simulink model "Longitudinal_Discrete_Servo_OutputFeedback"  (R2018b)
settings: Solver=VariableStepAuto  StartTime=0.0  StopTime=50  RelTol=1e-3
undefined symbols (not defined in the file): Gxd_A_obs, Gxd_B_obs, Gxd_C_obs, K0_X, K_X, KGe_X, t_samp
libraries: simulink x1
settings Model: Creator=Henrique  LastModifiedBy=Henrique

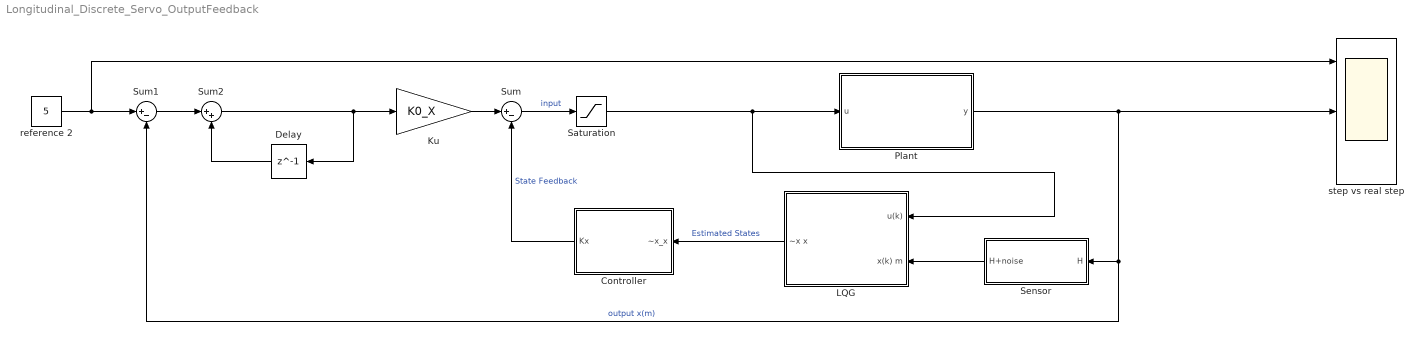
== system Longitudinal_Discrete_Servo_OutputFeedback ==
  "Controller " : Subsystem
  Delay : Delay  DelayLength=1  InitialCondition=0
  Ku : Gain  Gain=K0_X
  LQG : Subsystem
  Plant : Subsystem
  Saturation : Saturate  UpperLimit=2  LowerLimit=-1.2
  Sensor : Subsystem
  Sum : Sum  Inputs=|+-
  Sum1 : Sum  Inputs=|+-
  Sum2 : Sum  Inputs=|++
  reference 2 : Constant  Value=5
  "step vs real step " : Scope  NumInputPorts=3
  wires:
  LQG/1("~x x ") -> "Controller "/1(~x_x)  "Estimated States"
  Sum/1 -> Saturation/1  "input"
  "Controller "/1(Kx) -> Sum/2  "State Feedback"
  Plant/1("y ") -> "step vs real step "/2, Sensor/1(H), Sum1/2  "output x(m)"
  Saturation/1 -> Plant/1("u "), LQG/1(u(k))
  Sensor/1(H+noise) -> LQG/2(x(k) m)
  reference 2/1 -> Sum1/1, "step vs real step "/1
  Sum1/1 -> Sum2/1
  Sum2/1 -> Ku/1, Delay/1
  Ku/1 -> Sum/1
  Delay/1 -> Sum2/2

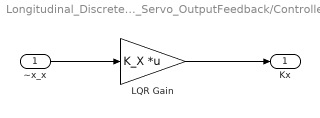
== system Longitudinal_Discrete_Servo_OutputFeedback/Controller  ==
  ~x_x : Inport
  "LQR Gain " : Gain  Gain=K_X  Multiplication=Matrix(K*u) (u vector)
  Kx : Outport
  wires:
  ~x_x/1 -> "LQR Gain "/1
  "LQR Gain "/1 -> Kx/1

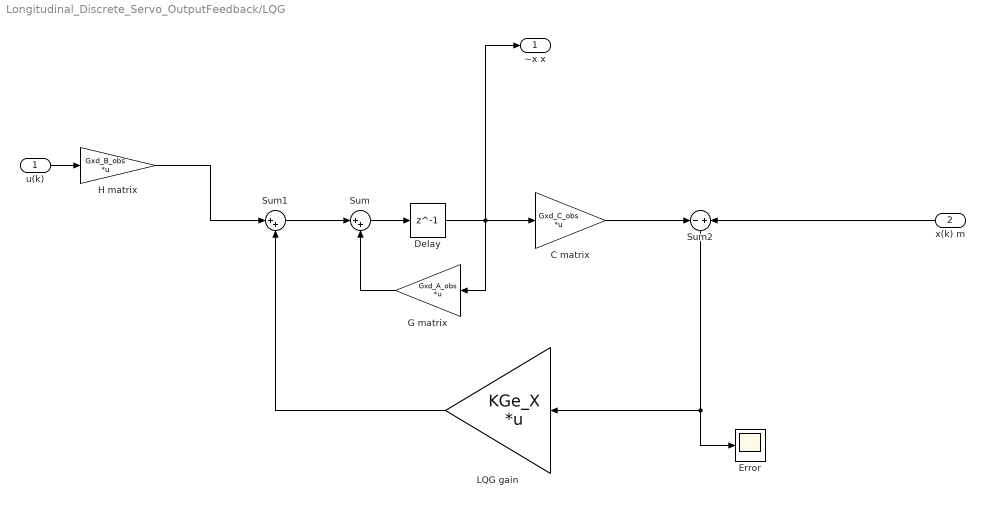
== system Longitudinal_Discrete_Servo_OutputFeedback/LQG ==
  u(k) : Inport
  x(k) m : Inport  Port=2
  C matrix : Gain  Gain=Gxd_C_obs  Multiplication=Matrix(K*u)
  Delay : Delay  DelayLength=1  InitialCondition=0  SampleTime=t_samp
  Error : Scope
  G matrix : Gain  Gain=Gxd_A_obs  Multiplication=Matrix(K*u)
  H matrix : Gain  Gain=Gxd_B_obs  Multiplication=Matrix(K*u)
  LQG gain : Gain  Gain=KGe_X  Multiplication=Matrix(K*u)
  Sum : Sum  Inputs=|++
  Sum1 : Sum  Inputs=|++
  Sum2 : Sum  Inputs=-+
  "~x x " : Outport
  wires:
  C matrix/1 -> Sum2/1
  x(k) m/1 -> Sum2/2
  H matrix/1 -> Sum1/1
  Sum/1 -> Delay/1
  u(k)/1 -> H matrix/1
  G matrix/1 -> Sum/2
  Sum2/1 -> Error/1, LQG gain/1
  LQG gain/1 -> Sum1/2
  Delay/1 -> "~x x "/1, G matrix/1, C matrix/1
  Sum1/1 -> Sum/1

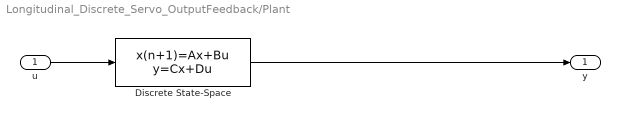
== system Longitudinal_Discrete_Servo_OutputFeedback/Plant ==
  "u " : Inport
  Discrete State-Space : DiscreteStateSpace  A=Gxd_A_obs  B=Gxd_B_obs  C=Gxd_C_obs  D=0  SampleTime=t_samp
  "y " : Outport
  wires:
  "u "/1 -> Discrete State-Space/1
  Discrete State-Space/1 -> "y "/1

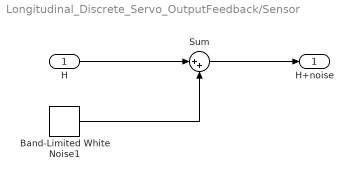
== system Longitudinal_Discrete_Servo_OutputFeedback/Sensor ==
  H : Inport
  Band-Limited White Noise1 : simulink/Sources/Band-Limited White Noise  Cov=.000001  Ts=0.1  seed=[124123]
  Sum : Sum  Inputs=|++
  H+noise : Outport
  wires:
  Sum/1 -> H+noise/1
  H/1 -> Sum/1
  Band-Limited White Noise1/1 -> Sum/2
